simulink model "pendule_simple"  (R2015a)
settings: Solver=ode3  StartTime=0.0  StopTime=10  FixedStep=0.01  RelTol=1e-3
undefined symbols (not defined in the file): l
libraries: simulink x1
settings Model: Creator=gmartini  LastModifiedBy=gregoire

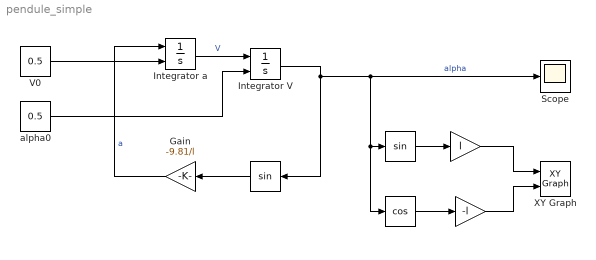
== system pendule_simple ==
  " " : Trigonometry
  " " : Trigonometry
  " " : Trigonometry  Operator=cos
  " " : Gain  Gain=-l
  " " : Gain  Gain=l
  Gain : Gain  Gain=-9.81/l
  Integrator V : Integrator  InitialConditionSource=external
  Integrator a : Integrator  InitialConditionSource=external
  Scope : Scope
      settings: YMin=-1  YMax=1
  V0 : Constant  Value=0.5
  XY Graph : simulink/Sinks/XY Graph  xmin=-1  xmax=1  ymin=-1  ymax=1  st=-1
  alpha0 : Constant  Value=0.5
  wires:
  Integrator a/1 -> Integrator V/1  "V"
  Integrator V/1 -> " "/1, " "/1, Scope/1, " "/1  "alpha"
  Gain/1 -> Integrator a/1  "a"
  " "/1 -> Gain/1
  V0/1 -> Integrator a/2
  " "/1 -> " "/1
  " "/1 -> " "/1
  " "/1 -> XY Graph/2
  " "/1 -> XY Graph/1
  alpha0/1 -> Integrator V/2
